simulink model "magnetic_dipole"  (R2024b)
settings: Solver=VariableStepAuto  StartTime=0.0  StopTime=10.0  RelTol=1e-3
undefined symbols (not defined in the file): WMM2020
libraries: aerolibtransform2 x1, aerolibgravity2 x1
settings Model: Creator=aditi  LastModifiedBy=aditi

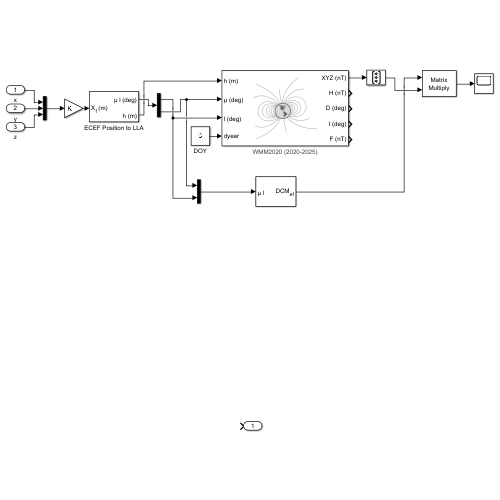
[thumbnail: Simulink's stored preview of the top-level diagram]
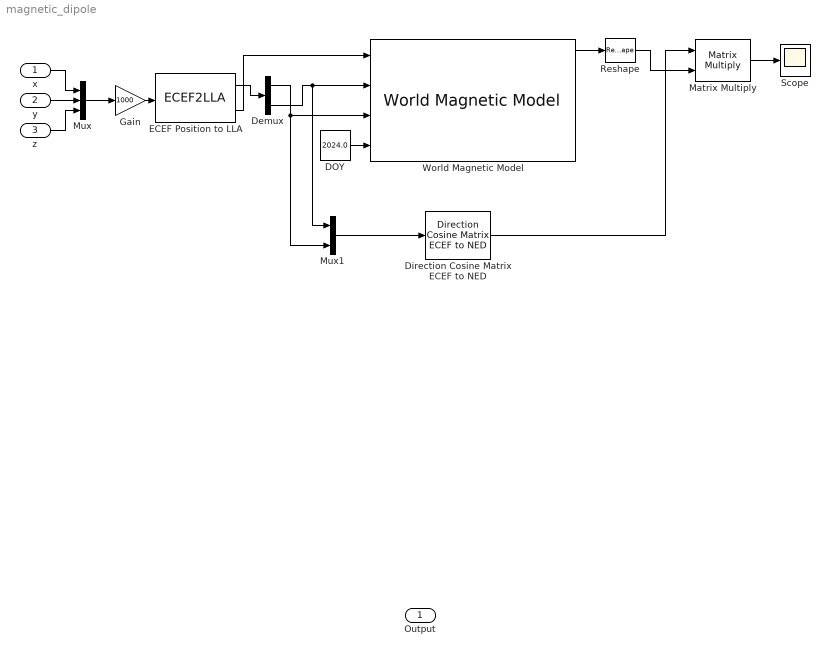
== system magnetic_dipole ==
  x : Inport  PortDimensions=1  LockScale=on
  y : Inport  Port=2  PortDimensions=1
  z : Inport  Port=3  PortDimensions=1
  DOY : Constant  Value=2024.0
  Demux : Demux  Outputs=2
  Direction Cosine Matrix ECEF to NED : aerolibtransform2/Direction Cosine Matrix ECEF to NED
  ECEF Position to LLA : ECEF2LLA
  Gain : Gain  Gain=1000
  Matrix Multiply : Product  Multiplication=Matrix(*)
  Mux : Mux  Inputs=3
  Mux1 : Mux  Inputs=2
  Reshape : Reshape  OutputDimensionality=Column vector (2-D)
  Scope : Scope
  World Magnetic Model : aerolibgravity2/World Magnetic Model  model=WMM2020 (2020-2025)  customFile='WMM2020.COF'  units=Metric (MKS)  time_in=on  month=January  day=1  year=2020  action=Error  h_out=on  dec_out=on  inc_out=on  ti_out=on
  Output : Outport
  wires:
  x/1 -> Mux/1
  y/1 -> Mux/2
  z/1 -> Mux/3
  ECEF Position to LLA/1 -> Demux/1
  Demux/1 -> Mux1/2, World Magnetic Model/3
  Demux/2 -> Mux1/1, World Magnetic Model/2
  DOY/1 -> World Magnetic Model/4
  World Magnetic Model/1 -> Reshape/1
  Matrix Multiply/1 -> Scope/1
  Mux1/1 -> Direction Cosine Matrix ECEF to NED/1
  Direction Cosine Matrix ECEF to NED/1 -> Matrix Multiply/1
  Reshape/1 -> Matrix Multiply/2
  Mux/1 -> Gain/1
  Gain/1 -> ECEF Position to LLA/1
  ECEF Position to LLA/2 -> World Magnetic Model/1
